simulink library "SoftRobotics_back"  (R2023b)
settings: Solver=VariableStepAuto  StartTime=0.0  StopTime=10.0  RelTol=1e-3
undefined symbols (not defined in the file or in its folder): bt, sr
settings Model: Creator=pietro  LastModifiedBy=pietro
settings OptimizationCC: ReuseModelBlockBuffer=off

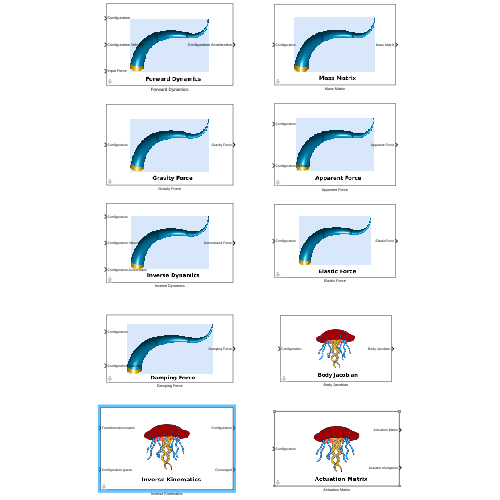
[thumbnail: Simulink's stored preview of the top-level diagram]
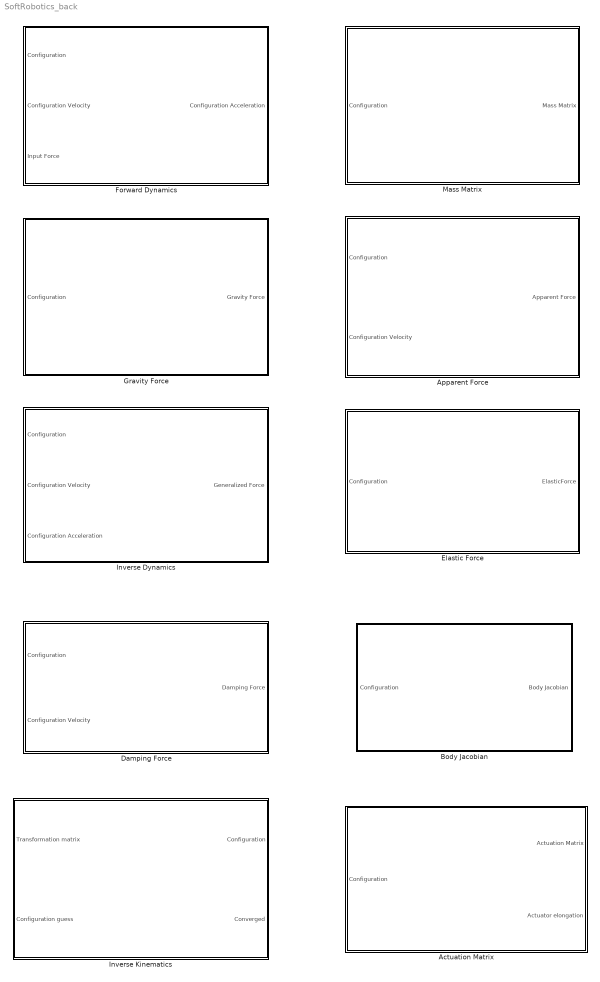
== system SoftRobotics_back ==
  Actuation Matrix : Subsystem  mask{robotModel=sr, SimulateUsing=Code generation}
      mask prompts: robotModel "Soft Robot Model"; SimulateUsing "SystemBlock:MATLABSystem:SimulateUsing"
      mask init:
      | %Get the robot representation as a struct (required for code generation)
      | Tree        = evalin('base', get_param(gcb, 'RobotModel'));
      | robotStruct = SoftRobotStructConverter.ObjectToStruct(Tree);
      | %Set the struct as a parameter of the underlying block
      | set_param([gcb '/' 'ActuationMatrixSystem'], 'SoftRobotStruct', 'robotStruct');
      mask TypeOptions SimulateUsing: ActuationMatrixSystem/SimulateUsing
      mask DialogControl SimulateUsing Prompt: Simulate using:
      mask DialogControl SimulateUsing Tooltip: SystemBlock:MATLABSystem:SimulateUsingDescription
  Apparent Force : Subsystem  mask{robotModel=bt, SimulateUsing=Code generation}
      mask prompts: robotModel "Robot Model"; SimulateUsing "SystemBlock:MATLABSystem:SimulateUsing"
      mask init:
      | %Get the robot representation as a struct (required for code generation)
      | Tree = evalin('base', get_param(gcb, 'RobotModel'));
      | robotStruct = TreeStructConverter.ObjectToStruct(Tree);
      | %Set the struct as a parameter of the underlying block
      | set_param([gcb '/' 'ApparentForceSystem'], 'RobotStruct', 'robotStruct');
      mask TypeOptions SimulateUsing: ApparentForceSystem/SimulateUsing
      mask DialogControl SimulateUsing Prompt: Simulate using:
      mask DialogControl SimulateUsing Tooltip: SystemBlock:MATLABSystem:SimulateUsingDescription
  Body Jacobian : Subsystem  mask{robotModel=bt, SimulateUsing=Code generation}
      mask prompts: robotModel "Robot Model"; SimulateUsing "SystemBlock:MATLABSystem:SimulateUsing"
      mask init:
      | %Get the robot representation as a struct (required for code generation)
      | Tree = evalin('base', get_param(gcb, 'RobotModel'));
      | robotStruct = TreeStructConverter.ObjectToStruct(Tree);
      | %Set the struct as a parameter of the underlying block
      | set_param([gcb '/' 'BodyJacobianSystem'], 'RobotStruct', 'robotStruct');
      mask TypeOptions SimulateUsing: BodyJacobianSystem/SimulateUsing
      mask DialogControl SimulateUsing Prompt: Simulate using:
      mask DialogControl SimulateUsing Tooltip: SystemBlock:MATLABSystem:SimulateUsingDescription
  Damping Force : Subsystem  mask{robotModel=bt, SimulateUsing=Code generation}
      mask prompts: robotModel "Robot Model"; SimulateUsing "SystemBlock:MATLABSystem:SimulateUsing"
      mask init:
      | %Get the robot representation as a struct (required for code generation)
      | Tree = evalin('base', get_param(gcb, 'RobotModel'));
      | robotStruct = TreeStructConverter.ObjectToStruct(Tree);
      | %Set the struct as a parameter of the underlying block
      | set_param([gcb '/' 'DampingForceSystem'], 'RobotStruct', 'robotStruct');
      mask TypeOptions SimulateUsing: DampingForceSystem/SimulateUsing
      mask DialogControl SimulateUsing Prompt: Simulate using:
      mask DialogControl SimulateUsing Tooltip: SystemBlock:MATLABSystem:SimulateUsingDescription
  Elastic Force : Subsystem  mask{robotModel=bt, SimulateUsing=Code generation}
      mask prompts: robotModel "Robot Model"; SimulateUsing "SystemBlock:MATLABSystem:SimulateUsing"
      mask init:
      | %Get the robot representation as a struct (required for code generation)
      | Tree = evalin('base', get_param(gcb, 'RobotModel'));
      | robotStruct = TreeStructConverter.ObjectToStruct(Tree);
      | %Set the struct as a parameter of the underlying block
      | set_param([gcb '/' 'ElasticForceSystem'], 'RobotStruct', 'robotStruct');
      mask TypeOptions SimulateUsing: ElasticForceSystem/SimulateUsing
      mask DialogControl SimulateUsing Prompt: Simulate using:
      mask DialogControl SimulateUsing Tooltip: SystemBlock:MATLABSystem:SimulateUsingDescription
  Forward Dynamics : Subsystem  mask{RobotModel=bt, SimulateUsing=Code generation}
      mask prompts: RobotModel "Robot model"; SimulateUsing "Simulate using:"
      mask init:
      | %TODO: Add various checks that the paramter is correct.
      | 
      | %Get the robot representation as a struct (required for code generation)
      | Tree = evalin('base', get_param(gcb, 'RobotModel'));
      | robotStruct = TreeStructConverter.ObjectToStruct(Tree);
      | %Set the struct as a parameter of the underlying block
      | set_param([gcb '/' 'ForwardDynamicsSystem'], 'RobotStruct', 'robotStruct');
      mask TypeOptions SimulateUsing: ForwardDynamicsSystem/SimulateUsing
      mask DialogControl DescTextVar Prompt: Implementazione delle forward dynamics
      mask DialogControl SimulateUsing Tooltip: SystemBlock:MATLABSystem:SimulateUsingDescription
  Gravity Force : Subsystem  mask{robotModel=bt, SimulateUsing=Code generation}
      mask prompts: robotModel "Robot Model"; SimulateUsing "SystemBlock:MATLABSystem:SimulateUsing"
      mask init:
      | %Get the robot representation as a struct (required for code generation)
      | Tree = evalin('base', get_param(gcb, 'RobotModel'));
      | robotStruct = TreeStructConverter.ObjectToStruct(Tree);
      | %Set the struct as a parameter of the underlying block
      | set_param([gcb '/' 'GravityForceSystem'], 'RobotStruct', 'robotStruct');
      mask TypeOptions SimulateUsing: GravityForceSystem/SimulateUsing
      mask DialogControl SimulateUsing Prompt: Simulate using:
      mask DialogControl SimulateUsing Tooltip: SystemBlock:MATLABSystem:SimulateUsingDescription
  Inverse Dynamics : Subsystem  mask{robotModel=bt, SimulateUsing=Code generation}
      mask prompts: robotModel "Robot Model"; SimulateUsing "SystemBlock:MATLABSystem:SimulateUsing"
      mask init:
      | %Get the robot representation as a struct (required for code generation)
      | Tree = evalin('base', get_param(gcb, 'RobotModel'));
      | robotStruct = TreeStructConverter.ObjectToStruct(Tree);
      | %Set the struct as a parameter of the underlying block
      | set_param([gcb '/' 'InverseDynamicsSystem'], 'RobotStruct', 'robotStruct');
      mask TypeOptions SimulateUsing: InverseDynamicsSystem/SimulateUsing
      mask DialogControl SimulateUsing Prompt: Simulate using:
      mask DialogControl SimulateUsing Tooltip: SystemBlock:MATLABSystem:SimulateUsingDescription
  Inverse Kinematics : Subsystem  mask{robotModel=bt, SimulateUsing=Code generation, BodyIndexes=1, MaximumNewtonIterations=4, TaskSpaceFlags=ones( 6, 1 )}
      mask prompts: robotModel "Robot Model"; SimulateUsing "SystemBlock:MATLABSystem:SimulateUsing"; BodyIndexes "Indexes of the bodies to consider in the inverse kinematics:"; MaximumNewtonIterations "Maximum number of Newton iterations:"; TaskSpaceFlags "Task space flags:"
      mask init:
      | %Get the robot representation as a struct (required for code generation)
      | Tree        = evalin('base', get_param(gcb, 'RobotModel'));
      | robotStruct = TreeStructConverter.ObjectToStruct(Tree);
      | %Set the struct as a parameter of the underlying block
      | set_param([gcb '/' 'InverseKinematicsSystem'], 'RobotStruct', 'robotStruct');
      mask TypeOptions SimulateUsing: InverseKinematicsSystem/SimulateUsing
      mask TypeOptions BodyIndexes: InverseKinematicsSystem/BodyIndexes
      mask TypeOptions MaximumNewtonIterations: InverseKinematicsSystem/MaximumNewtonIterations
      mask TypeOptions TaskSpaceFlags: InverseKinematicsSystem/TaskSpaceFlags
      mask DialogControl SimulateUsing Prompt: Simulate using:
      mask DialogControl SimulateUsing Tooltip: SystemBlock:MATLABSystem:SimulateUsingDescription
  Mass Matrix : Subsystem  mask{RobotModel=bt, SimulateUsing=Code generation}
      mask prompts: RobotModel "Robot model"; SimulateUsing "SystemBlock:MATLABSystem:SimulateUsing"
      mask init:
      | %Get the robot representation as a struct (required for code generation)
      | Tree = evalin('base', get_param(gcb, 'RobotModel'));
      | robotStruct = TreeStructConverter.ObjectToStruct(Tree);
      | %Set the struct as a parameter of the underlying block
      | set_param([gcb '/' 'MassMatrixSystem'], 'RobotStruct', 'robotStruct');
      mask TypeOptions SimulateUsing: MassMatrixSystem/SimulateUsing
      mask DialogControl SimulateUsing Prompt: Simulate using:
      mask DialogControl SimulateUsing Tooltip: SystemBlock:MATLABSystem:SimulateUsingDescription

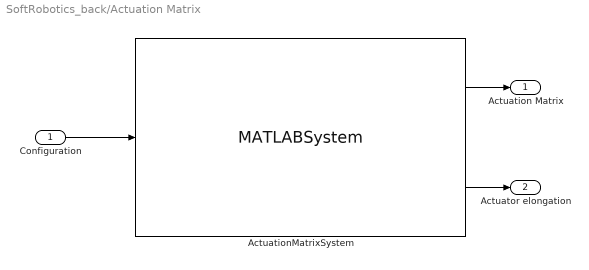
== system SoftRobotics_back/Actuation Matrix ==
  Configuration : Inport
  ActuationMatrixSystem : MATLABSystem  System=ActuationMatrixSystem  SoftRobotStruct=0  SimulateUsing=Code generation
      mask Type: ActuationMatrixSystem
      mask Display:
      | disp('ActuationMatrixSystem');
      | port_label('input',1,'q');
      | port_label('output',1,'A');
      | port_label('output',2,'y');
  Actuation Matrix : Outport
  Actuator elongation : Outport  Port=2
  wires:
  ActuationMatrixSystem/1 -> Actuation Matrix/1
  Configuration/1 -> ActuationMatrixSystem/1
  ActuationMatrixSystem/2 -> Actuator elongation/1

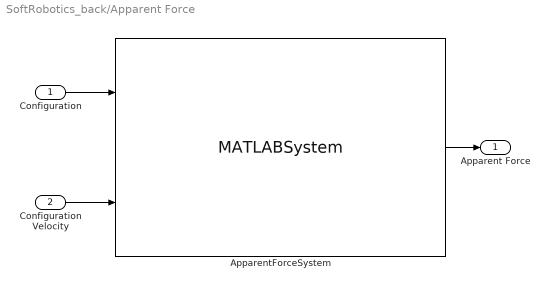
== system SoftRobotics_back/Apparent Force ==
  Configuration : Inport
  Configuration Velocity : Inport  Port=2
  ApparentForceSystem : MATLABSystem  System=ApparentForceSystem  RobotStruct=robotStruct  SimulateUsing=Code generation
      mask Type: ApparentForceSystem
      mask Display:
      | disp('ApparentForceSystem');
      | port_label('input',1,'q');
      | port_label('input',2,'dq');
      | port_label('output',1,'C');
  Apparent Force : Outport
  wires:
  Configuration Velocity/1 -> ApparentForceSystem/2
  ApparentForceSystem/1 -> Apparent Force/1
  Configuration/1 -> ApparentForceSystem/1

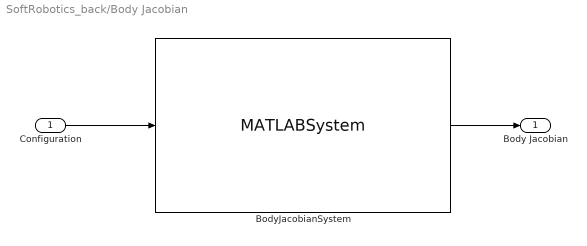
== system SoftRobotics_back/Body Jacobian ==
  Configuration : Inport
  BodyJacobianSystem : MATLABSystem  System=BodyJacobianSystem  RobotStruct=bt  SimulateUsing=Code generation
      mask Type: BodyJacobianSystem
      mask Display:
      | disp('BodyJacobianSystem');
      | port_label('input',1,'q');
      | port_label('output',1,'J');
  Body Jacobian : Outport
  wires:
  Configuration/1 -> BodyJacobianSystem/1
  BodyJacobianSystem/1 -> Body Jacobian/1

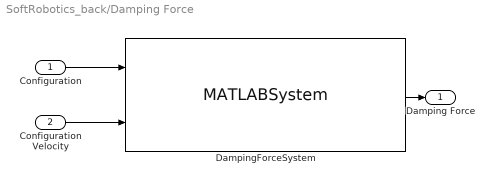
== system SoftRobotics_back/Damping Force ==
  Configuration : Inport
  Configuration Velocity : Inport  Port=2
  DampingForceSystem : MATLABSystem  System=DampingForceSystem  RobotStruct=robotStruct  SimulateUsing=Code generation
      mask Type: DampingForceSystem
      mask Display:
      | disp('DampingForceSystem');
      | port_label('input',1,'q');
      | port_label('input',2,'dq');
      | port_label('output',1,'D');
  Damping Force : Outport
  wires:
  Configuration/1 -> DampingForceSystem/1
  DampingForceSystem/1 -> Damping Force/1
  Configuration Velocity/1 -> DampingForceSystem/2

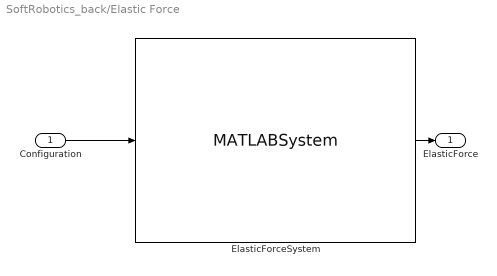
== system SoftRobotics_back/Elastic Force ==
  Configuration : Inport
  ElasticForceSystem : MATLABSystem  System=ElasticForceSystem  RobotStruct=robotStruct  SimulateUsing=Code generation
      mask Type: ElasticForceSystem
      mask Display:
      | disp('ElasticForceSystem');
      | port_label('input',1,'q');
      | port_label('output',1,'K');
  ElasticForce : Outport
  wires:
  Configuration/1 -> ElasticForceSystem/1
  ElasticForceSystem/1 -> ElasticForce/1

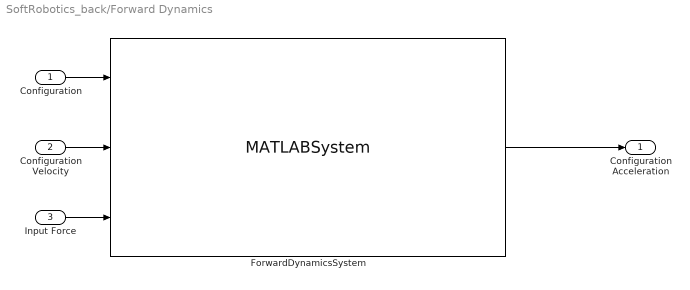
== system SoftRobotics_back/Forward Dynamics ==
  Configuration : Inport
  Configuration Velocity : Inport  Port=2
  Input Force : Inport  Port=3
  ForwardDynamicsSystem : MATLABSystem  System=ForwardDynamicsSystem  RobotStruct=robotStruct  SimulateUsing=Code generation
      mask Type: ForwardDynamicsSystem
      mask Display:
      | disp('ForwardDynamicsSystem');
      | port_label('input',1,'q');
      | port_label('input',2,'dq');
      | port_label('input',3,'u');
      | port_label('output',1,'ddq');
  Configuration Acceleration : Outport
  wires:
  Configuration/1 -> ForwardDynamicsSystem/1
  Configuration Velocity/1 -> ForwardDynamicsSystem/2
  Input Force/1 -> ForwardDynamicsSystem/3
  ForwardDynamicsSystem/1 -> Configuration Acceleration/1

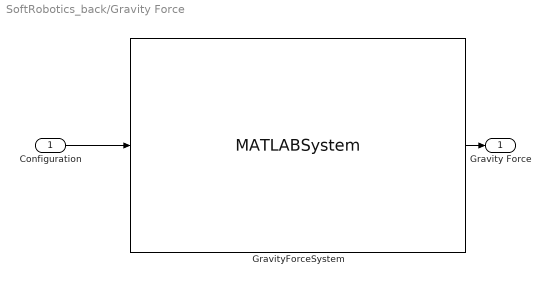
== system SoftRobotics_back/Gravity Force ==
  Configuration : Inport
  GravityForceSystem : MATLABSystem  System=GravityForceSystem  RobotStruct=robotStruct  SimulateUsing=Code generation
      mask Type: GravityForceSystem
      mask Display:
      | disp('GravityForceSystem');
      | port_label('input',1,'q');
      | port_label('output',1,'G');
  Gravity Force : Outport
  wires:
  Configuration/1 -> GravityForceSystem/1
  GravityForceSystem/1 -> Gravity Force/1

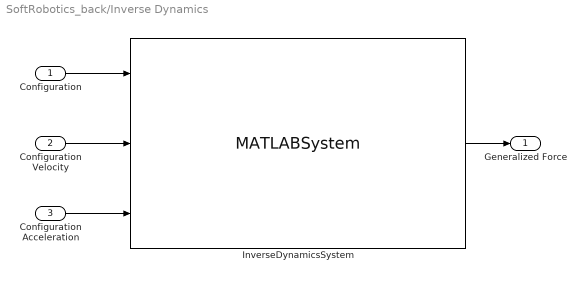
== system SoftRobotics_back/Inverse Dynamics ==
  Configuration : Inport
  Configuration Velocity : Inport  Port=2
  Configuration Acceleration : Inport  Port=3
  InverseDynamicsSystem : MATLABSystem  System=InverseDynamicsSystem  RobotStruct=robotStruct  SimulateUsing=Code generation
      mask Type: InverseDynamicsSystem
      mask Display:
      | disp('InverseDynamicsSystem');
      | port_label('input',1,'q');
      | port_label('input',2,'dq');
      | port_label('input',3,'ddq');
      | port_label('output',1,'u');
  Generalized Force : Outport
  wires:
  Configuration Velocity/1 -> InverseDynamicsSystem/2
  InverseDynamicsSystem/1 -> Generalized Force/1
  Configuration/1 -> InverseDynamicsSystem/1
  Configuration Acceleration/1 -> InverseDynamicsSystem/3

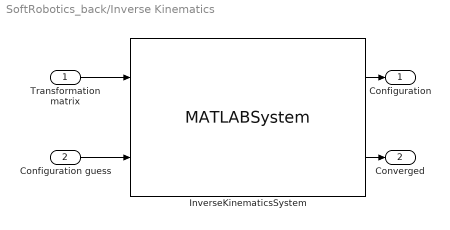
== system SoftRobotics_back/Inverse Kinematics ==
  Transformation matrix : Inport
  Configuration guess : Inport  Port=2
  InverseKinematicsSystem : MATLABSystem  System=InverseKinematicsSystem  RobotStruct=0  BodyIndexes=BodyIndexes  MaximumNewtonIterations=MaximumNewtonIterations  TaskSpaceFlags=TaskSpaceFlags  SimulateUsing=Code generation
      mask Type: InverseKinematicsSystem
      mask Display:
      | disp('InverseKinematicsSystem');
      | port_label('input',1,'T');
      | port_label('input',2,'q0');
      | port_label('output',1,'q');
      | port_label('output',2,'converged');
  Configuration : Outport
  Converged : Outport  Port=2
  wires:
  Configuration guess/1 -> InverseKinematicsSystem/2
  InverseKinematicsSystem/1 -> Configuration/1
  Transformation matrix/1 -> InverseKinematicsSystem/1
  InverseKinematicsSystem/2 -> Converged/1

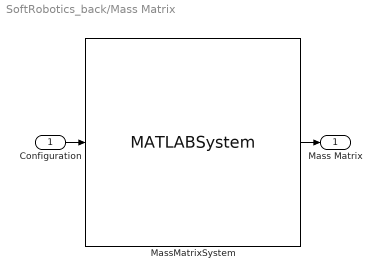
== system SoftRobotics_back/Mass Matrix ==
  Configuration : Inport
  MassMatrixSystem : MATLABSystem  System=MassMatrixSystem  RobotStruct=robotStruct  SimulateUsing=Code generation
      mask Type: MassMatrixSystem
      mask Display:
      | disp('MassMatrixSystem');
      | port_label('input',1,'q');
      | port_label('output',1,'M');
  Mass Matrix : Outport
  wires:
  Configuration/1 -> MassMatrixSystem/1
  MassMatrixSystem/1 -> Mass Matrix/1
